simulink model "bilant_termic"  (R2021a)
settings: Solver=VariableStepAuto  StartTime=0.0  StopTime=10.0  RelTol=1e-3
values from neighbouring files (symbols this model uses):
  hA = kT*At    (= 18821.555234)    [script.m]
  mdH = 24953    [script.m]
  rcp = 2093    [script.m]
  T0 = 339.437    [script.m]
  V = 10    [script.m]
settings Model: Creator=Automatica  LastModifiedBy=Automatica

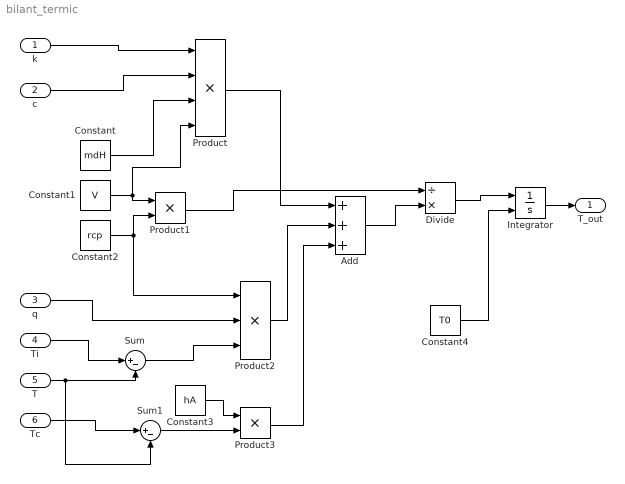
== system bilant_termic ==
  k : Inport
  c : Inport  Port=2
  q : Inport  Port=3
  Ti : Inport  Port=4
  T : Inport  Port=5
  Tc : Inport  Port=6
  Add : Sum  Inputs=+++
  Constant : Constant  Value=mdH
  Constant1 : Constant  Value=V
  Constant2 : Constant  Value=rcp
  Constant3 : Constant  Value=hA
  Constant4 : Constant  Value=T0
  Divide : Product  Inputs=/*
  Integrator : Integrator  InitialConditionSource=external
  Product : Product  Inputs=4
  Product1 : Product
  Product2 : Product  Inputs=3
  Product3 : Product
  Sum : Sum  Inputs=|+-
  Sum1 : Sum  Inputs=|+-
  T_out : Outport
  wires:
  k/1 -> Product/1
  c/1 -> Product/2
  Constant/1 -> Product/3
  Constant1/1 -> Product1/1, Product/4
  Constant2/1 -> Product2/1, Product1/2
  q/1 -> Product2/2
  Tc/1 -> Sum1/1
  T/1 -> Sum1/2, Sum/2
  Ti/1 -> Sum/1
  Sum/1 -> Product2/3
  Sum1/1 -> Product3/2
  Constant3/1 -> Product3/1
  Product3/1 -> Add/3
  Product2/1 -> Add/2
  Product/1 -> Add/1
  Product1/1 -> Divide/1
  Add/1 -> Divide/2
  Divide/1 -> Integrator/1
  Constant4/1 -> Integrator/2
  Integrator/1 -> T_out/1
